simulink library "ddm"  (R2021b)
settings: Solver=VariableStepAuto  StartTime=0.0  StopTime=10.0  RelTol=1e-3
undefined symbols (not defined in the file or in its folder): ENUM_ADASACCSTA_ERROR, ENUM_ADASACCSTA_OFF, ENUM_ADASACCSTA_STANDBY, ENUM_ADASISASTA_OFF, ENUM_ALLOWMOV_ALLOWREADY, ENUM_APS, ENUM_BRKSTA_ERROR, ENUM_BRKSTA_OFF, ENUM_BRKSTA_ON, ENUM_BRKSW_INVALID, ENUM_BRKSW_OFF, ENUM_BRKSW_ON, ENUM_CHGPREACTERRSTA_OBCPRE, ENUM_DCDCFAULTSTA_ANYFAULTLV1, ENUM_DCDCFAULTSTA_ANYFAULTLV2, ENUM_DRIVETRAIN_AWD, ENUM_DRIVETRAIN_FWD, ENUM_DRIVETRAIN_RWD, ENUM_DRSEATSTA_INVALID, ENUM_EDUDRTSTA_NORMAL, ENUM_EPBSTA_APPLIED, ENUM_EPBSTA_RELEASED, ENUM_HVBATTREADYPRE_READY, ENUM_MCUWARN_LV0, ENUM_MCUWARN_LV1, ENUM_MCUWARN_LV2, ENUM_MCUWARN_LV3, ENUM_MCUWARN_NOERROR, ENUM_OBCFAULTSTA_ANYFAULT, ENUM_PAS_R2F2, ENUM_PDFAULT_BATTPDFAIL, ENUM_PDFAULT_DCDCDISABLE, ENUM_PDFAULT_MCUDISABLE, ENUM_PDFAULT_MCUDISCHRG, ENUM_POWERSTA_OFF, ENUM_POWERSTA_ON, ENUM_POWERSTA_READY, ENUM_POWERSTA_STANDBY, ENUM_PRESSINDI_LOW, ENUM_PUFAULT_BATTUPFAIL, ENUM_PUFAULT_DCDCENABLEFAIL, ENUM_PUFAULT_PRECHRGCHKFAIL, ENUM_PUFAULT_SAFETYCHKFAIL, ENUM_PUSTATE_COMPLETED, ENUM_PWRSTASW_OFF, ENUM_PWRSTASW_OFFA, ENUM_PWRSTASW_OFFCHVCHRG, ENUM_PWRSTASW_OFFCLVCHRG, ENUM_PWRSTASW_ON, ENUM_PWRSTASW_ONHVCHRG, ENUM_PWRSTASW_READY, ENUM_PWRSTASW_STANDBY, ENUM_RANGESTA_12IN, ENUM_SHIFTCOMMAND_D, ENUM_SHIFTCOMMAND_N, ENUM_SHIFTCOMMAND_P, ENUM_SHIFTCOMMAND_R, ENUM_VEHMALFUNLV_2ND, ENUM_VEHMALFUNLV_3RD, ENUM_VEHMALFUNLV_4TH ... (+835)
libraries: hcu_lib x750, $bdroot x12, simulink x5
(part 27 of 28)

== system ddm/DDM/DDM/VMC_DDM/MCU_Rr Signal Error/MCU_Rr Signal Error  ==
  note: Diagnostics and Fault Handling
  note: Fail Safe After Decision
  note: Release Condiction During Detection
  note: Release Condiction After Decision
  note: Test Pass Criteria
  note: Test Detection Criteria
  note: Fail Safe During Detection
  task_time_s : Inport
  VDDM_MCUF1NoComCFS_flg : Inport  Port=2
  VDDM_MCUF1RCErrCFS_flg : Inport  Port=3
  VDDM_MCUF1CSErrCFS_flg : Inport  Port=4
  No_CAN_BUS_OFF : Inport  Port=5
  VPMM_PowerSta_enum : Inport  Port=6
  VINP_MCUWarnR_enum : Inport  Port=7
  DTC_clear_request : Inport  Port=8
  Constant : Constant  Value=ENUM_POWERSTA_OFF
  Constant1 : Constant  Value=ENUM_POWERSTA_OFF
  Constant10 : Constant  Value=ENUM_MCUWARN_LV3
  Constant11 : Constant  Value=KDDM_RrMCUSigErrPassSW_flg
  Constant12 : Constant  Value=ENUM_POWERSTA_OFF
  Constant13 : Constant  Value=ENUM_POWERSTA_STANDBY
  Constant{5,14,18,22} (4 alike) : Constant  Value=TRUE
  Constant{2,15,20..21,23} (5 alike) : Constant  Value=FALSE
  Constant16 : Constant  Value=ENUM_MCUWARN_LV3
  Constant17 : Constant  Value=ENUM_MCUWARN_LV1
  Constant19 : Constant  Value=ENUM_MCUWARN_LV2
  Constant3 : Constant  Value=ENUM_MCUWARN_LV1
  Constant33 : Constant  Value=KDDM_RrMCUSigErrDetSW_flg
  Constant34 : Constant  Value=KDDM_RrMCUSigErrDTC_cnt
  Constant35 : Constant  Value=KDDM_RrMCUSigErrCFSSW_flg
  Constant36 : Constant  Value=KDDM_RrMCUSigErrDFSSW_flg
  Constant4 : Constant  Value=KDDM_RrMCUSigErrDetTO_ms
  Constant6 : Constant  Value=KDDM_RrMCUSigErrPassTO_ms
  Constant7 : Constant  Value=KDDM_RrMCUSigErrDTC_cnt
  Constant8 : Constant  Value=ENUM_MCUWARN_LV2
  Constant9 : Constant  Value=KDDM_RrMCUSigErrPassTO_ms
  DTC_Couter : hcu_lib/Basic_Blocks/DTC_Couter
  DTC_Info : hcu_lib/Basic_Blocks/DTC_Info
  Data Type Conversion1 : DataTypeConversion  OutDataTypeStr=uint8
  Equal : RelationalOperator  Operator=~=  OutDataTypeStr=boolean  RndMeth=Simplest
  Equal1 : RelationalOperator  Operator=~=  OutDataTypeStr=boolean  RndMeth=Simplest
  Equal{2,4..10} (8 alike) : RelationalOperator  Operator===  OutDataTypeStr=boolean  RndMeth=Simplest
  Equal3 : RelationalOperator  OutDataTypeStr=boolean  RndMeth=Simplest
  From1 : From  Commented=on  GotoTag=VDDM_RrMCUSigErrDFS_flg
  Gain : Gain  Gain=XX2KXX
  Gain1 : Gain  Gain=KXX2XX
  Goto7 : Goto  Commented=on  GotoTag=VDDM_EDriveSysErrVCUErr_flg
  Logical Operator{1,7..8,16,25} (5 alike) : Logic  Operator=OR  Inputs=3  AllPortsSameDT=off  OutDataTypeStr=boolean
  Logical Operator10 : Logic  Operator=OR  AllPortsSameDT=off  OutDataTypeStr=boolean
  Logical Operator{3,5,9,15} (4 alike) : Logic  AllPortsSameDT=off  OutDataTypeStr=boolean
  Logical Operator{4,6,17..18,20..22,24} (8 alike) : Logic  Operator=NOT  AllPortsSameDT=off  OutDataTypeStr=boolean
  Logical Operator19 : Logic  Inputs=3  AllPortsSameDT=off  OutDataTypeStr=boolean
  Logical Operator2 : Logic  Inputs=5  AllPortsSameDT=off  OutDataTypeStr=boolean
  Logical Operator23 : Logic  Inputs=5  AllPortsSameDT=off  OutDataTypeStr=boolean
  Relay : Relay  OnSwitchValue=ONE_INT  OffSwitchValue=ZERO_INT
  SR_Latch1 : hcu_lib/Basic_Blocks/SR_Latch
  SR_Latch4 : hcu_lib/Basic_Blocks/SR_Latch
  SR_Latch5 : hcu_lib/Basic_Blocks/SR_Latch
  Switch{,1..5} (6 alike) : Switch  Criteria=u2 ~= 0
  Terminator1 : Terminator
  Test Detection Criteria : hcu_lib/Basic_Blocks/Test Detection Criteria
  Timer1 : hcu_lib/Basic_Blocks/Timer
  Unit Delay2 : UnitDelay  SampleTime=-1  HasFrameUpgradeWarning=on
  VDDM_RrMCUSigErrCFS_flg : Outport
  VDDM_RrMCUSigErrDetDTC_raw32 : Outport  Port=2
  wires:
  Logical Operator15/1 -> DTC_Couter/2
  [DTC_clear_request] -> Logical Operator25/1, Logical Operator4/1
  Constant11/1 -> Logical Operator15/2
  [VDDM_RrMCUSigErrDet_flg] -> Logical Operator19/1
  Constant34/1 -> DTC_Couter/3
  [VDDM_RrMCUSigErrDTC_cnt] -> Relay/1
  Constant33/1 -> Logical Operator19/2
  [DTC_clear_request] -> Logical Operator7/3
  Logical Operator4/1 -> Logical Operator19/3
  Logical Operator10/1 -> SR_Latch5/2
  [VDDM_RrMCUSigErrDFSRls_flg] -> Logical Operator7/1
  DTC_Couter/2 -> Data Type Conversion1/1
  Data Type Conversion1/1 -> [VDDM_RrMCUSigErrDTC_cnt]
  Constant36/1 -> Logical Operator3/1
  SR_Latch5/1 -> Logical Operator5/1
  Logical Operator19/1 -> DTC_Couter/1
  SR_Latch4/1 -> Logical Operator3/2
  [VDDM_RrMCUSigErrCFSRls_flg] -> Logical Operator10/1
  [VDDM_RrMCUSigErrCFS_flg] -> Logical Operator7/2
  Constant35/1 -> Logical Operator5/2
  [VDDM_RrMCUSigErrCFSRls_flg] -> Logical Operator25/3
  Logical Operator7/1 -> SR_Latch4/2
  [VDDM_RrMCUSigErrPass_flg] -> Logical Operator25/2
  Logical Operator3/1 -> [VDDM_RrMCUSigErrDFS_flg]
  Logical Operator5/1 -> [VDDM_RrMCUSigErrCFS_flg]  "VDDM_RrMCUSigErrCFS_flg"
  [DTC_clear_request] -> Logical Operator10/2
  Logical Operator25/1 -> Logical Operator15/1
  DTC_Couter/1 -> SR_Latch5/1
  Relay/1 -> SR_Latch4/1
  DTC_Info/1 -> VDDM_RrMCUSigErrDetDTC_raw32/1  "VDDM_RrMCUSigErrDetDTC_raw32"
  [DTC_clear_request] -> DTC_Info/4
  [VDDM_RrMCUSigErrCFS_flg] -> DTC_Info/3
  [VDDM_RrMCUSigErrPass_flg] -> DTC_Info/2
  [VDDM_RrMCUSigErrDet_flg] -> DTC_Info/1
  Switch5/1 -> Test Detection Criteria/1
  Constant20/1 -> Switch5/1
  [DTC_clear_request] -> Switch5/2
  [VINP_MCUWarnR_enum] -> Equal10/1
  Constant16/1 -> Equal10/2
  [VINP_MCUWarnR_enum] -> Equal8/1
  Logical Operator1/1 -> Switch3/1
  Constant17/1 -> Equal8/2
  Equal8/1 -> Logical Operator1/1
  Equal9/1 -> Logical Operator1/2
  Equal10/1 -> Logical Operator1/3
  Constant19/1 -> Equal9/2
  [VINP_MCUWarnR_enum] -> Equal9/1
  Equal5/1 -> Logical Operator16/3
  Equal4/1 -> Logical Operator16/2
  Equal2/1 -> Logical Operator16/1
  Constant10/1 -> Equal5/2
  [VINP_MCUWarnR_enum] -> Equal5/1
  [VINP_MCUWarnR_enum] -> Equal4/1
  Constant8/1 -> Equal4/2
  Constant3/1 -> Equal2/2
  Constant9/1 -> Timer1/4
  Gain1/1 -> Timer1/3
  Test Detection Criteria/1 -> [VDDM_RrMCUSigErrDet_flg]  "VDDM_RrMCUSigErrDet_flg"
  Constant7/1 -> Test Detection Criteria/3
  Gain/1 -> Test Detection Criteria/4
  Constant4/1 -> Gain/1
  [task_time_s] -> Test Detection Criteria/2
  task_time_s/1 -> [task_time_s]  "task_time_s"
  Switch3/1 -> Logical Operator6/1, Timer1/2
  Constant1/1 -> Equal1/2
  [No_CAN_BUS_OFF] -> Logical Operator23/1
  [VDDM_MCUF1CSErrCFS_flg] -> Logical Operator24/1
  Logical Operator21/1 -> Logical Operator23/2
  Logical Operator24/1 -> Logical Operator23/4
  [VDDM_MCUF1RCErrCFS_flg] -> Logical Operator22/1
  Equal1/1 -> Logical Operator23/5
  Constant5/1 -> Switch3/3
  Logical Operator23/1 -> Switch3/2
  [VPMM_PowerSta_enum] -> Equal1/1
  [VDDM_MCUF1NoComCFS_flg] -> Logical Operator21/1
  Logical Operator22/1 -> Logical Operator23/3
  Logical Operator20/1 -> Logical Operator2/4
  Logical Operator18/1 -> Logical Operator2/3
  Logical Operator17/1 -> Logical Operator2/2
  [VINP_MCUWarnR_enum] -> Equal2/1
  Logical Operator16/1 -> Switch2/1
  [VDDM_MCUF1CSErrCFS_flg] -> Logical Operator20/1
  [VDDM_MCUF1RCErrCFS_flg] -> Logical Operator18/1
  [VDDM_MCUF1NoComCFS_flg] -> Logical Operator17/1
  Equal/1 -> Logical Operator2/5
  VINP_MCUWarnR_enum/1 -> [VINP_MCUWarnR_enum]
  No_CAN_BUS_OFF/1 -> [No_CAN_BUS_OFF]
  VDDM_MCUF1CSErrCFS_flg/1 -> [VDDM_MCUF1CSErrCFS_flg]
  VPMM_PowerSta_enum/1 -> [VPMM_PowerSta_enum]
  VDDM_MCUF1RCErrCFS_flg/1 -> [VDDM_MCUF1RCErrCFS_flg]
  DTC_clear_request/1 -> [DTC_clear_request]
  VDDM_MCUF1NoComCFS_flg/1 -> [VDDM_MCUF1NoComCFS_flg]
  Timer1/1 -> Equal3/1
  [VPMM_PowerSta_enum] -> Equal/1
  Logical Operator8/1 -> Switch4/2
  [VPMM_PowerSta_enum] -> Equal7/1
  Constant14/1 -> Switch4/1
  Constant2/1 -> Switch2/3
  Constant12/1 -> Equal6/2
  Unit Delay2/1 -> Equal6/1
  Constant/1 -> Equal/2
  Constant13/1 -> Equal7/2
  Logical Operator6/1 -> Timer1/1
  Logical Operator2/1 -> Switch2/2
  [DTC_clear_request] -> Logical Operator8/3
  [VDDM_xxx_flg] -> SR_Latch1/2
  [VDDM_RrMCUSigErrPass_flg] -> Logical Operator8/1
  [No_CAN_BUS_OFF] -> Logical Operator2/1
  Switch4/1 -> [VDDM_RrMCUSigErrCFSRls_flg]  "VDDM_RrMCUSigErrCFSRls_flg"
  Logical Operator9/1 -> Logical Operator8/2
  [VPMM_PowerSta_enum] -> Unit Delay2/1
  Constant6/1 -> Equal3/2
  Equal7/1 -> Logical Operator9/2
  Equal6/1 -> Logical Operator9/1
  [task_time_s] -> Gain1/1
  Equal3/1 -> SR_Latch1/1
  Constant15/1 -> Switch4/3
  [VDDM_RrMCUSigErrCFS_flg] -> VDDM_RrMCUSigErrCFS_flg/1
  From1/1 -> Terminator1/1
  SR_Latch1/1 -> [VDDM_RrMCUSigErrPass_flg]  "VDDM_RrMCUSigErrPass_flg"
  [VDDM_RrMCUSigErrPass_flg] -> Switch1/2
  [VDDM_RrMCUSigErrCFS_flg] -> Switch/2
  Constant18/1 -> Switch/1
  Switch/1 -> Goto7/1
  Constant21/1 -> Switch/3
  Switch1/1 -> [VDDM_RrMCUSigErrDFSRls_flg]
  Constant22/1 -> Switch1/1
  Constant23/1 -> Switch1/3
  Switch2/1 -> Switch5/3, [VDDM_xxx_flg]

== system ddm/DDM/DDM/VMC_DDM/MSA Malfunction /MSA Malfunction ==
  note: Diagnostics and Fault Handling
  note: Fail Safe After Decision
  note: Release Condiction During Detection
  note: Release Condiction After Decision
  note: Test Pass Criteria
  note: Test Detection Criteria
  note: Fail Safe During Detection
  task_time_s : Inport
  VDDM_BMSSigErrCFS_flg : Inport  Port=2
  VDDM_FrMCUSigErrCFS_flg : Inport  Port=3
  VDDM_RrMCUSigErrCFS_flg : Inport  Port=4
  VDDM_CCUSigErrCFS_flg : Inport  Port=5
  VDDM_ZoneSCPNoComCFS_flg : Inport  Port=6
  VDDM_MCUR1NoComCFS_flg : Inport  Port=7
  VDDM_MCUR1RCErrCFS_flg : Inport  Port=8
  VDDM_MCUR1CSErrCFS_flg : Inport  Port=9
  VDDM_MCUF1NoComCFS_flg : Inport  Port=10
  VDDM_MCUF1RCErrCFS_flg : Inport  Port=11
  VDDM_MCUF1CSErrCFS_flg : Inport  Port=12
  VDDM_ESC7NoComCFS_flg : Inport  Port=13
  VDDM_ESC7RCErrCFS_flg : Inport  Port=14
  VDDM_ESC7CSErrCFS_flg : Inport  Port=15
  VDDM_ESC1NoComCFS_flg : Inport  Port=16
  VDDM_ESC1RCErrCFS_flg : Inport  Port=17
  VDDM_ESC1CSErrCFS_flg : Inport  Port=18
  VDDM_ESC5NoComCFS_flg : Inport  Port=19
  VDDM_ESC5RCErrCFS_flg : Inport  Port=20
  VDDM_ESC5CSErrCFS_flg : Inport  Port=21
  No_CAN1_BUS_OFF : Inport  Port=22
  No_CAN3_BUS_OFF : Inport  Port=23
  No_CAN4_BUS_OFF : Inport  Port=24
  VPMM_PowerSta_enum : Inport  Port=25
  VINP_ZoneSpdCtrlMode_enum : Inport  Port=26
  DTC_clear_request : Inport  Port=27
  Constant1 : Constant  Value=ENUM_POWERSTA_READY
  Constant10 : Constant  Value=ENUM_ZONESPDCTRLMODE_LIM
  Constant11 : Constant  Value=KDDM_MSAMalfuncPassSW_flg
  Constant12 : Constant  Value=ENUM_POWERSTA_OFF
  Constant13 : Constant  Value=ENUM_POWERSTA_STANDBY
  Constant{5,14,18,22} (4 alike) : Constant  Value=TRUE
  Constant{2,15..16,21,23} (5 alike) : Constant  Value=FALSE
  Constant3 : Constant  Value=ENUM_ZONESPDCTRLMODE_LIM
  Constant33 : Constant  Value=KDDM_MSAMalfuncDetSW_flg
  Constant34 : Constant  Value=KDDM_MSAMalfuncDTC_cnt
  Constant35 : Constant  Value=KDDM_MSAMalfuncCFSSW_flg
  Constant36 : Constant  Value=KDDM_MSAMalfuncDFSSW_flg
  Constant4 : Constant  Value=KDDM_MSAMalfuncDetTO_ms
  Constant6 : Constant  Value=KDDM_MSAMalfuncPassTO_ms
  Constant7 : Constant  Value=KDDM_MSAMalfuncDTC_cnt
  Constant8 : Constant  Value=ENUM_POWERSTA_READY
  Constant9 : Constant  Value=KDDM_MSAMalfuncPassTO_ms
  DTC_Couter : hcu_lib/Basic_Blocks/DTC_Couter
  DTC_Info : hcu_lib/Basic_Blocks/DTC_Info
  Data Type Conversion1 : DataTypeConversion  OutDataTypeStr=uint8
  Equal{1..2,4..7} (6 alike) : RelationalOperator  Operator===  OutDataTypeStr=boolean  RndMeth=Simplest
  Equal3 : RelationalOperator  OutDataTypeStr=boolean  RndMeth=Simplest
  From1 : From  Commented=on  GotoTag=VDDM_MSAMalfuncDFS_flg
  Gain : Gain  Gain=XX2KXX
  Gain1 : Gain  Gain=KXX2XX
  Goto7 : Goto  Commented=on  GotoTag=VDDM_EDriveSysErrVCUErr_flg
  Logical Operator1 : Logic  Inputs=5  AllPortsSameDT=off  OutDataTypeStr=boolean
  Logical Operator12 : Logic  Operator=OR  Inputs=3  AllPortsSameDT=off  OutDataTypeStr=boolean
  Logical Operator{3,5,13,15} (4 alike) : Logic  AllPortsSameDT=off  OutDataTypeStr=boolean
  Logical Operator14 : Logic  Operator=OR  Inputs=20  AllPortsSameDT=off  OutDataTypeStr=boolean
  Logical Operator19 : Logic  Inputs=3  AllPortsSameDT=off  OutDataTypeStr=boolean
  Logical Operator2 : Logic  Inputs=5  AllPortsSameDT=off  OutDataTypeStr=boolean
  Logical Operator25 : Logic  Operator=OR  Inputs=3  AllPortsSameDT=off  OutDataTypeStr=boolean
  Logical Operator4 : Logic  Operator=OR  Inputs=20  AllPortsSameDT=off  OutDataTypeStr=boolean
  Logical Operator6 : Logic  Operator=NOT  AllPortsSameDT=off  OutDataTypeStr=boolean
  Logical Operator7 : Logic  Operator=OR  Inputs=3  AllPortsSameDT=off  OutDataTypeStr=boolean
  Logical Operator8 : Logic  Operator=NOT  AllPortsSameDT=off  OutDataTypeStr=boolean
  Logical Operator9 : Logic  Operator=OR  AllPortsSameDT=off  OutDataTypeStr=boolean
  Relay : Relay  OnSwitchValue=ONE_INT  OffSwitchValue=ZERO_INT
  SR_Latch1 : hcu_lib/Basic_Blocks/SR_Latch
  SR_Latch4 : hcu_lib/Basic_Blocks/SR_Latch
  SR_Latch5 : hcu_lib/Basic_Blocks/SR_Latch
  Switch{,1..5} (6 alike) : Switch  Criteria=u2 ~= 0
  Terminator1 : Terminator
  Test Detection Criteria : hcu_lib/Basic_Blocks/Test Detection Criteria
  Timer1 : hcu_lib/Basic_Blocks/Timer
  Unit Delay2 : UnitDelay  SampleTime=-1  HasFrameUpgradeWarning=on
  VDDM_MSAMalfuncCFS_flg : Outport
  VDDM_MSAMalfuncDetDTC_raw32 : Outport  Port=2
  wires:
  SR_Latch5/1 -> Logical Operator5/1
  [DTC_clear_request] -> Logical Operator7/3
  [DTC_clear_request] -> Logical Operator25/1, Logical Operator8/1
  Data Type Conversion1/1 -> [VDDM_MSAMalfuncDTC_cnt]  "VDDM_MSAMalfuncDTC_cnt"
  Logical Operator5/1 -> [VDDM_MSAMalfuncCFS_flg]  "VDDM_MSAMalfuncCFS_flg"
  Logical Operator8/1 -> Logical Operator19/3
  Constant35/1 -> Logical Operator5/2
  [VDDM_MSAMalfuncDTC_cnt] -> Relay/1
  SR_Latch4/1 -> Logical Operator3/2
  Logical Operator25/1 -> Logical Operator15/1
  Logical Operator15/1 -> DTC_Couter/2
  [VDDM_MSAMalfuncDFSRls_flg] -> Logical Operator7/1
  Logical Operator3/1 -> [VDDM_MSAMalfuncDFS_flg]
  Constant11/1 -> Logical Operator15/2
  [DTC_clear_request] -> Logical Operator9/2
  Logical Operator7/1 -> SR_Latch4/2
  Relay/1 -> SR_Latch4/1
  [VDDM_MSAMalfuncDet_flg] -> Logical Operator19/1
  DTC_Couter/2 -> Data Type Conversion1/1
  [VDDM_MSAMalfuncPass_flg] -> Logical Operator25/2
  [VDDM_MSAMalfuncCFSRls_flg] -> Logical Operator25/3
  Logical Operator19/1 -> DTC_Couter/1
  Constant34/1 -> DTC_Couter/3
  Constant33/1 -> Logical Operator19/2
  DTC_Couter/1 -> SR_Latch5/1
  [VDDM_MSAMalfuncCFSRls_flg] -> Logical Operator9/1
  Constant36/1 -> Logical Operator3/1
  [VDDM_MSAMalfuncCFS_flg] -> Logical Operator7/2
  Logical Operator9/1 -> SR_Latch5/2
  DTC_Info/1 -> VDDM_MSAMalfuncDetDTC_raw32/1  "VDDM_MSAMalfuncDetDTC_raw32"
  [DTC_clear_request] -> DTC_Info/4
  [VDDM_MSAMalfuncCFS_flg] -> DTC_Info/3
  [VDDM_MSAMalfuncPass_flg] -> DTC_Info/2
  [VDDM_MSAMalfuncDet_flg] -> DTC_Info/1
  Switch5/1 -> Test Detection Criteria/1
  Constant16/1 -> Switch5/1
  [DTC_clear_request] -> Switch5/2
  [VDDM_ESC5CSErrCFS_flg] -> Logical Operator4/20
  [VDDM_MCUR1CSErrCFS_flg] -> Logical Operator4/8
  [VDDM_ESC5NoComCFS_flg] -> Logical Operator4/18
  Logical Operator4/1 -> Switch3/1
  [VDDM_CCUSigErrCFS_flg] -> Logical Operator4/4
  [VDDM_MCUR1RCErrCFS_flg] -> Logical Operator4/7
  [VDDM_ESC1CSErrCFS_flg] -> Logical Operator4/17
  [VDDM_MCUF1NoComCFS_flg] -> Logical Operator4/9
  [VDDM_MCUR1NoComCFS_flg] -> Logical Operator4/6
  [VDDM_MCUF1CSErrCFS_flg] -> Logical Operator4/11
  [VDDM_MCUF1RCErrCFS_flg] -> Logical Operator4/10
  [VDDM_ESC7NoComCFS_flg] -> Logical Operator4/12
  [VDDM_ESC1NoComCFS_flg] -> Logical Operator4/15
  [VDDM_ESC7RCErrCFS_flg] -> Logical Operator4/13
  [VDDM_ESC5RCErrCFS_flg] -> Logical Operator4/19
  [VDDM_ESC7CSErrCFS_flg] -> Logical Operator4/14
  [VDDM_BMSSigErrCFS_flg] -> Logical Operator4/1
  [VDDM_FrMCUSigErrCFS_flg] -> Logical Operator4/2
  [VDDM_RrMCUSigErrCFS_flg] -> Logical Operator4/3
  [VDDM_ZoneSCPNoComCFS_flg] -> Logical Operator4/5
  [VDDM_ESC1RCErrCFS_flg] -> Logical Operator4/16
  [VDDM_ESC5CSErrCFS_flg] -> Logical Operator14/20
  [VDDM_ESC5RCErrCFS_flg] -> Logical Operator14/19
  [VDDM_ESC5NoComCFS_flg] -> Logical Operator14/18
  [VDDM_ESC1CSErrCFS_flg] -> Logical Operator14/17
  [VDDM_ESC1RCErrCFS_flg] -> Logical Operator14/16
  [VDDM_ESC1NoComCFS_flg] -> Logical Operator14/15
  [VDDM_ESC7CSErrCFS_flg] -> Logical Operator14/14
  [VDDM_ESC7RCErrCFS_flg] -> Logical Operator14/13
  [VDDM_ESC7NoComCFS_flg] -> Logical Operator14/12
  [VDDM_MCUF1CSErrCFS_flg] -> Logical Operator14/11
  [VDDM_MCUF1RCErrCFS_flg] -> Logical Operator14/10
  [VDDM_MCUF1NoComCFS_flg] -> Logical Operator14/9
  [VDDM_MCUR1CSErrCFS_flg] -> Logical Operator14/8
  [VDDM_MCUR1RCErrCFS_flg] -> Logical Operator14/7
  [VDDM_MCUR1NoComCFS_flg] -> Logical Operator14/6
  [VDDM_ZoneSCPNoComCFS_flg] -> Logical Operator14/5
  [VDDM_CCUSigErrCFS_flg] -> Logical Operator14/4
  [VDDM_RrMCUSigErrCFS_flg] -> Logical Operator14/3
  [VDDM_FrMCUSigErrCFS_flg] -> Logical Operator14/2
  [VDDM_BMSSigErrCFS_flg] -> Logical Operator14/1
  Logical Operator1/1 -> Switch3/2
  [No_CAN1_BUS_OFF] -> Logical Operator1/1
  [No_CAN3_BUS_OFF] -> Logical Operator1/2
  Equal4/1 -> Logical Operator1/5
  Equal5/1 -> Logical Operator1/4
  Constant8/1 -> Equal5/2
  Constant10/1 -> Equal4/2
  [VPMM_PowerSta_enum] -> Equal5/1
  [No_CAN4_BUS_OFF] -> Logical Operator1/3
  [VINP_ZoneSpdCtrlMode_enum] -> Equal4/1
  Equal1/1 -> Logical Operator2/5
  Constant3/1 -> Equal1/2
  [VINP_ZoneSpdCtrlMode_enum] -> Equal1/1
  [VPMM_PowerSta_enum] -> Equal2/1
  Constant1/1 -> Equal2/2
  Equal2/1 -> Logical Operator2/4
  [No_CAN4_BUS_OFF] -> Logical Operator2/3
  [No_CAN3_BUS_OFF] -> Logical Operator2/2
  Logical Operator14/1 -> Switch2/1
  VDDM_ESC5RCErrCFS_flg/1 -> [VDDM_ESC5RCErrCFS_flg]
  VDDM_ESC5CSErrCFS_flg/1 -> [VDDM_ESC5CSErrCFS_flg]
  VDDM_ESC5NoComCFS_flg/1 -> [VDDM_ESC5NoComCFS_flg]
  VDDM_ZoneSCPNoComCFS_flg/1 -> [VDDM_ZoneSCPNoComCFS_flg]
  task_time_s/1 -> [task_time_s]  "task_time_s"
  VINP_ZoneSpdCtrlMode_enum/1 -> [VINP_ZoneSpdCtrlMode_enum]
  No_CAN3_BUS_OFF/1 -> [No_CAN3_BUS_OFF]
  No_CAN1_BUS_OFF/1 -> [No_CAN1_BUS_OFF]
  VDDM_BMSSigErrCFS_flg/1 -> [VDDM_BMSSigErrCFS_flg]
  VDDM_ESC7NoComCFS_flg/1 -> [VDDM_ESC7NoComCFS_flg]
  VDDM_ESC7CSErrCFS_flg/1 -> [VDDM_ESC7CSErrCFS_flg]
  VPMM_PowerSta_enum/1 -> [VPMM_PowerSta_enum]
  No_CAN4_BUS_OFF/1 -> [No_CAN4_BUS_OFF]
  VDDM_ESC7RCErrCFS_flg/1 -> [VDDM_ESC7RCErrCFS_flg]
  VDDM_RrMCUSigErrCFS_flg/1 -> [VDDM_RrMCUSigErrCFS_flg]
  VDDM_CCUSigErrCFS_flg/1 -> [VDDM_CCUSigErrCFS_flg]
  VDDM_FrMCUSigErrCFS_flg/1 -> [VDDM_FrMCUSigErrCFS_flg]
  VDDM_MCUF1RCErrCFS_flg/1 -> [VDDM_MCUF1RCErrCFS_flg]
  VDDM_ESC1NoComCFS_flg/1 -> [VDDM_ESC1NoComCFS_flg]
  DTC_clear_request/1 -> [DTC_clear_request]
  VDDM_MCUR1RCErrCFS_flg/1 -> [VDDM_MCUR1RCErrCFS_flg]
  VDDM_MCUR1CSErrCFS_flg/1 -> [VDDM_MCUR1CSErrCFS_flg]
  VDDM_ESC1RCErrCFS_flg/1 -> [VDDM_ESC1RCErrCFS_flg]
  VDDM_ESC1CSErrCFS_flg/1 -> [VDDM_ESC1CSErrCFS_flg]
  VDDM_MCUF1CSErrCFS_flg/1 -> [VDDM_MCUF1CSErrCFS_flg]
  VDDM_MCUF1NoComCFS_flg/1 -> [VDDM_MCUF1NoComCFS_flg]
  VDDM_MCUR1NoComCFS_flg/1 -> [VDDM_MCUR1NoComCFS_flg]
  [VDDM_MSAMalfuncPass_flg] -> Logical Operator12/1
  Constant12/1 -> Equal6/2
  Constant13/1 -> Equal7/2
  Equal6/1 -> Logical Operator13/1
  Logical Operator13/1 -> Logical Operator12/2
  Equal7/1 -> Logical Operator13/2
  Unit Delay2/1 -> Equal6/1
  [VPMM_PowerSta_enum] -> Equal7/1
  [VPMM_PowerSta_enum] -> Unit Delay2/1
  Constant9/1 -> Timer1/4
  Gain1/1 -> Timer1/3
  Test Detection Criteria/1 -> [VDDM_MSAMalfuncDet_flg]  "VDDM_MSAMalfuncDet_flg"
  Constant7/1 -> Test Detection Criteria/3
  Gain/1 -> Test Detection Criteria/4
  Constant4/1 -> Gain/1
  [task_time_s] -> Test Detection Criteria/2
  Switch3/1 -> Logical Operator6/1, Timer1/2
  Constant5/1 -> Switch3/3
  Timer1/1 -> Equal3/1
  Logical Operator12/1 -> Switch4/2
  Constant14/1 -> Switch4/1
  Constant2/1 -> Switch2/3
  Logical Operator6/1 -> Timer1/1
  Logical Operator2/1 -> Switch2/2
  [DTC_clear_request] -> Logical Operator12/3
  [VDDM_xxx_flg] -> SR_Latch1/2
  [No_CAN1_BUS_OFF] -> Logical Operator2/1
  Switch4/1 -> [VDDM_MSAMalfuncCFSRls_flg]  "VDDM_MSAMalfuncCFSRls_flg"
  Constant6/1 -> Equal3/2
  [task_time_s] -> Gain1/1
  Equal3/1 -> SR_Latch1/1
  Constant15/1 -> Switch4/3
  [VDDM_MSAMalfuncCFS_flg] -> VDDM_MSAMalfuncCFS_flg/1
  From1/1 -> Terminator1/1
  SR_Latch1/1 -> [VDDM_MSAMalfuncPass_flg]  "VDDM_MSAMalfuncPass_flg"
  [VDDM_MSAMalfuncPass_flg] -> Switch1/2
  [VDDM_MSAMalfuncCFS_flg] -> Switch/2
  Constant18/1 -> Switch/1
  Switch/1 -> Goto7/1
  Constant21/1 -> Switch/3
  Switch1/1 -> [VDDM_MSAMalfuncDFSRls_flg]
  Constant22/1 -> Switch1/1
  Constant23/1 -> Switch1/3
  Switch2/1 -> Switch5/3, [VDDM_xxx_flg]

== system ddm/DDM/DDM/VMC_DDM/ZoneSCP/ZoneSCP Lost Com ==
  note: Diagnostics and Fault Handling
  note: Fail Safe During Detection
  note: Test Detection Criteria
  note: Release Condiction After Decision
  note: Test Pass Criteria
  note: Release Condiction During Detection
  note: Fail Safe After Decision
  task_time_s : Inport
  VDDM_ZoneSCPNoCom_flg : Inport  Port=2
  No_CAN_BUS_OFF : Inport  Port=3
  VPMM_PowerSta_enum : Inport  Port=4
  VINP_VehSpeed_kph : Inport  Port=5
  DTC_clear_request : Inport  Port=6
  Constant : Constant  Value=ENUM_POWERSTA_OFF
  Constant1 : Constant  Value=KDDM_ZoneSCPNoComCFSRls_kph
  Constant12 : Constant  Value=ENUM_POWERSTA_OFF
  Constant13 : Constant  Value=ENUM_POWERSTA_STANDBY
  Constant{7,14,18,22} (4 alike) : Constant  Value=TRUE
  Constant{2,8,15,21,23} (5 alike) : Constant  Value=FALSE
  Constant3 : Constant  Value=KDDM_ZoneSCPNoComDFSRls_kph
  Constant31 : Constant  Value=KDDM_ZoneSCPNoComDFSSW_flg
  Constant4 : Constant  Value=KDDM_ZoneSCPNoComCFSSW_flg
  Constant40 : Constant  Value=KDDM_ZoneSCPNoComDTC_cnt
  Constant41 : Constant  Value=KDDM_ZoneSCPNoComDetTO_ms
  Constant45 : Constant  Value=KDDM_ZoneSCPNoComPassSW_flg
  Constant46 : Constant  Value=KDDM_ZoneSCPNoComDetSW_flg
  Constant48 : Constant  Value=KDDM_ZoneSCPNoComDTC_cnt
  Constant5 : Constant  Value=ENUM_POWERSTA_OFF
  Constant6 : Constant  Value=KDDM_ZoneSCPNoComPassTO_ms
  Constant9 : Constant  Value=KDDM_ZoneSCPNoComPassTO_ms
  DTC_Couter : hcu_lib/Basic_Blocks/DTC_Couter
  DTC_Info : hcu_lib/Basic_Blocks/DTC_Info
  Data Type Conversion1 : DataTypeConversion  OutDataTypeStr=uint8
  Equal : RelationalOperator  Operator=~=  OutDataTypeStr=boolean  RndMeth=Simplest
  Equal1 : RelationalOperator  Operator=<=  OutDataTypeStr=boolean  RndMeth=Simplest
  Equal2 : RelationalOperator  Operator=~=  OutDataTypeStr=boolean  RndMeth=Simplest
  Equal3 : RelationalOperator  OutDataTypeStr=boolean  RndMeth=Simplest
  Equal4 : RelationalOperator  Operator=<=  OutDataTypeStr=boolean  RndMeth=Simplest
  Equal6 : RelationalOperator  Operator===  OutDataTypeStr=boolean  RndMeth=Simplest
  Equal7 : RelationalOperator  Operator===  OutDataTypeStr=boolean  RndMeth=Simplest
  From6 : From  Commented=on  GotoTag=VDDM_EDriveSysErrVCUErr_flg
  Gain : Gain  Gain=XX2KXX
  Gain1 : Gain  Gain=KXX2XX
  Goto7 : Goto  Commented=on  GotoTag=VDDM_EDriveSysErrVCUErr_flg
  Logical Operator{1..2,4..5,9,12,15,18} (8 alike) : Logic  AllPortsSameDT=off  OutDataTypeStr=boolean
  Logical Operator10 : Logic  Operator=OR  AllPortsSameDT=off  OutDataTypeStr=boolean
  Logical Operator19 : Logic  Inputs=3  AllPortsSameDT=off  OutDataTypeStr=boolean
  Logical Operator21 : Logic  Operator=OR  Inputs=3  AllPortsSameDT=off  OutDataTypeStr=boolean
  Logical Operator3 : Logic  Operator=OR  Inputs=3  AllPortsSameDT=off  OutDataTypeStr=boolean
  Logical Operator6 : Logic  Operator=NOT  AllPortsSameDT=off  OutDataTypeStr=boolean
  Logical Operator7 : Logic  Operator=NOT  AllPortsSameDT=off  OutDataTypeStr=boolean
  Logical Operator8 : Logic  Operator=OR  Inputs=3  AllPortsSameDT=off  OutDataTypeStr=boolean
  Relay : Relay  OnSwitchValue=ONE_INT  OffSwitchValue=ZERO_INT
  SR_Latch1 : hcu_lib/Basic_Blocks/SR_Latch
  SR_Latch3 : hcu_lib/Basic_Blocks/SR_Latch
  SR_Latch4 : hcu_lib/Basic_Blocks/SR_Latch
  Switch{,1..5} (6 alike) : Switch  Criteria=u2 ~= 0
  Terminator : Terminator
  Test Detection Criteria : hcu_lib/Basic_Blocks/Test Detection Criteria
  Timer1 : hcu_lib/Basic_Blocks/Timer
  Unit Delay2 : UnitDelay  SampleTime=-1  HasFrameUpgradeWarning=on
  VDDM_ZoneSCPNoComDFS_flg : Outport
  VDDM_ZoneSCPNoComCFS_flg : Outport  Port=2
  VDDM_ZoneSCPNoComDTC_raw32 : Outport  Port=3
  wires:
  Logical Operator3/1 -> Logical Operator15/1
  Logical Operator7/1 -> Logical Operator19/3
  [DTC_clear_request] -> Logical Operator21/3
  Constant48/1 -> DTC_Couter/3
  Logical Operator10/1 -> SR_Latch4/2
  DTC_Couter/2 -> Data Type Conversion1/1
  [DTC_clear_request] -> Logical Operator10/2
  SR_Latch3/1 -> Logical Operator12/2
  [DTC_clear_request] -> Logical Operator3/1, Logical Operator7/1
  Logical Operator15/1 -> DTC_Couter/2
  SR_Latch4/1 -> Logical Operator18/1
  Constant45/1 -> Logical Operator15/2
  Constant31/1 -> Logical Operator12/1
  [VDDM_ZoneSCPNoComDet_flg] -> Logical Operator19/1
  Logical Operator21/1 -> SR_Latch3/2
  Logical Operator12/1 -> [VDDM_ZoneSCPNoComDFS_flg]  "VDDM_ZoneSCPNoComDFS_flg"
  Relay/1 -> SR_Latch3/1
  [VDDM_ZoneSCPNoComCFS_flg] -> Logical Operator21/2
  Data Type Conversion1/1 -> [VDDM_ZoneSCPNoComDTC_cnt]
  [VDDM_ZoneSCPNoComCFSRls_flg] -> Logical Operator3/3
  Logical Operator18/1 -> [VDDM_ZoneSCPNoComCFS_flg]  "VDDM_ZoneSCPNoComCFS_flg"
  [VDDM_ZoneSCPNoComCFSRls_flg] -> Logical Operator10/1
  Constant4/1 -> Logical Operator18/2
  [VDDM_ZoneSCPNoComDTC_cnt] -> Relay/1
  [VDDM_ZoneSCPNoComPass_flg] -> Logical Operator3/2
  [VDDM_ZoneSCPNoComDFSRls_flg] -> Logical Operator21/1
  Constant46/1 -> Logical Operator19/2
  DTC_Couter/1 -> SR_Latch4/1
  Logical Operator19/1 -> DTC_Couter/1
  DTC_Info/1 -> VDDM_ZoneSCPNoComDTC_raw32/1  "VDDM_ZoneSCPNoComDTC_raw32"
  [DTC_clear_request] -> DTC_Info/4
  [VDDM_ZoneSCPNoComCFS_flg] -> DTC_Info/3
  [VDDM_ZoneSCPNoComPass_flg] -> DTC_Info/2
  [VDDM_ZoneSCPNoComDet_flg] -> DTC_Info/1
  Switch5/1 -> Test Detection Criteria/1
  [DTC_clear_request] -> Switch5/2
  Constant8/1 -> Switch5/1
  Equal4/1 -> Logical Operator1/2
  [VDDM_ZoneSCPNoComPass_flg] -> Logical Operator1/1
  Logical Operator1/1 -> Switch1/2
  [VINP_VehSpeed_kph] -> Equal4/1
  Constant3/1 -> Equal4/2
  Constant1/1 -> Equal1/2
  [VINP_VehSpeed_kph] -> Equal1/1
  Equal1/1 -> Logical Operator5/2
  Gain1/1 -> Timer1/3
  Constant9/1 -> Timer1/4
  task_time_s/1 -> [task_time_s]  "task_time_s"
  Constant40/1 -> Test Detection Criteria/3
  Constant6/1 -> Equal3/2
  SR_Latch1/1 -> [VDDM_ZoneSCPNoComPass_flg]  "VDDM_ZoneSCPNoComPass_flg"
  Gain/1 -> Test Detection Criteria/4
  Equal/1 -> Logical Operator2/2
  [VDDM_ZoneSCPNoComPass_flg] -> Logical Operator5/1
  Equal2/1 -> Logical Operator4/2
  [No_CAN_BUS_OFF] -> Logical Operator4/1
  Logical Operator9/1 -> Logical Operator8/2
  Logical Operator8/1 -> Switch4/2
  [VPMM_PowerSta_enum] -> Equal7/1
  [VPMM_PowerSta_enum] -> Equal2/1
  [VDDM_ZoneSCPNoCom_flg] -> Switch3/1
  Switch2/1 -> Switch5/3, [VDDM_xxx_flg]
  Constant/1 -> Equal/2
  Switch3/1 -> Timer1/2, Logical Operator6/1
  [VPMM_PowerSta_enum] -> Equal/1
  Switch4/1 -> [VDDM_ZoneSCPNoComCFSRls_flg]  "VDDM_ZoneSCPNoComCFSRls_flg"
  Constant41/1 -> Gain/1
  [task_time_s] -> Test Detection Criteria/2
  Test Detection Criteria/1 -> [VDDM_ZoneSCPNoComDet_flg]  "VDDM_ZoneSCPNoComDet_flg"
  Logical Operator2/1 -> Switch2/2
  Constant23/1 -> Switch1/3
  Timer1/1 -> Equal3/1
  Constant21/1 -> Switch/3
  Equal7/1 -> Logical Operator9/2
  [VDDM_ZoneSCPNoCom_flg] -> Switch2/1
  Logical Operator5/1 -> Logical Operator8/1
  Constant7/1 -> Switch3/3
  Logical Operator4/1 -> Switch3/2
  Constant14/1 -> Switch4/1
  Constant2/1 -> Switch2/3
  Constant12/1 -> Equal6/2
  Unit Delay2/1 -> Equal6/1
  [DTC_clear_request] -> Logical Operator8/3
  Constant5/1 -> Equal2/2
  Switch/1 -> Goto7/1
  Switch1/1 -> [VDDM_ZoneSCPNoComDFSRls_flg]  "VDDM_ZoneSCPNoComDFSRls_flg"
  Equal3/1 -> SR_Latch1/1
  Constant18/1 -> Switch/1
  Constant13/1 -> Equal7/2
  Equal6/1 -> Logical Operator9/1
  [task_time_s] -> Gain1/1
  Constant15/1 -> Switch4/3
  [VPMM_PowerSta_enum] -> Unit Delay2/1
  [VDDM_ZoneSCPNoComCFS_flg] -> Switch/2
  [No_CAN_BUS_OFF] -> Logical Operator2/1
  [VDDM_xxx_flg] -> SR_Latch1/2
  Constant22/1 -> Switch1/1
  Logical Operator6/1 -> Timer1/1
  From6/1 -> Terminator/1
  [VDDM_ZoneSCPNoComDFS_flg] -> VDDM_ZoneSCPNoComDFS_flg/1
  [VDDM_ZoneSCPNoComCFS_flg] -> VDDM_ZoneSCPNoComCFS_flg/1
  VDDM_ZoneSCPNoCom_flg/1 -> [VDDM_ZoneSCPNoCom_flg]
  VINP_VehSpeed_kph/1 -> [VINP_VehSpeed_kph]
  No_CAN_BUS_OFF/1 -> [No_CAN_BUS_OFF]
  DTC_clear_request/1 -> [DTC_clear_request]
  VPMM_PowerSta_enum/1 -> [VPMM_PowerSta_enum]

== system ddm/DDM/DDM/PMM/Brake switch signal abnormal/Brake switch signal abnormal/SR_Latch1 ==
  set : Inport
  reset : Inport  Port=2
  Logical Operator : Logic  AllPortsSameDT=off  OutDataTypeStr=boolean
  Logical Operator1 : Logic  Operator=NOT  AllPortsSameDT=off  OutDataTypeStr=boolean
  Switch1 : Switch  Criteria=u2 ~= 0  Threshold=0.5
      settings: AttributesFormatString=<Criteria=%<Criteria>>
  Switch2 : Switch  Criteria=u2 ~= 0  Threshold=0.5
      settings: AttributesFormatString=<Criteria=%<Criteria>>
  Unit Delay : UnitDelay  SampleTime=-1  HasFrameUpgradeWarning=on
  latched : Outport
  wires:
  Logical Operator1/1 -> Switch2/1, Logical Operator/2
  Logical Operator/1 -> Switch1/2
  Switch2/1 -> Switch1/3
  Unit Delay/1 -> Switch2/3
  reset/1 -> Logical Operator1/1, Switch2/2
  set/1 -> Logical Operator/1, Switch1/1
  Switch1/1 -> latched/1, Unit Delay/1

== system ddm/DDM/DDM/PMM/Brake switch signal abnormal/Brake switch signal abnormal and no backup signal/SR_Latch1 ==
  set : Inport
  reset : Inport  Port=2
  Logical Operator : Logic  AllPortsSameDT=off  OutDataTypeStr=boolean
  Logical Operator1 : Logic  Operator=NOT  AllPortsSameDT=off  OutDataTypeStr=boolean
  Switch1 : Switch  Criteria=u2 ~= 0  Threshold=0.5
      settings: AttributesFormatString=<Criteria=%<Criteria>>
  Switch2 : Switch  Criteria=u2 ~= 0  Threshold=0.5
      settings: AttributesFormatString=<Criteria=%<Criteria>>
  Unit Delay : UnitDelay  SampleTime=-1  HasFrameUpgradeWarning=on
  latched : Outport
  wires:
  Logical Operator1/1 -> Switch2/1, Logical Operator/2
  Logical Operator/1 -> Switch1/2
  Switch2/1 -> Switch1/3
  Unit Delay/1 -> Switch2/3
  reset/1 -> Logical Operator1/1, Switch2/2
  set/1 -> Logical Operator/1, Switch1/1
  Switch1/1 -> latched/1, Unit Delay/1

== system ddm/DDM/DDM/PMM/Comm err/FDC lost communication with EPAS2/SR_Latch1 ==
  set : Inport
  reset : Inport  Port=2
  Logical Operator : Logic  AllPortsSameDT=off  OutDataTypeStr=boolean
  Logical Operator1 : Logic  Operator=NOT  AllPortsSameDT=off  OutDataTypeStr=boolean
  Switch1 : Switch  Criteria=u2 ~= 0  Threshold=0.5
      settings: AttributesFormatString=<Criteria=%<Criteria>>
  Switch2 : Switch  Criteria=u2 ~= 0  Threshold=0.5
      settings: AttributesFormatString=<Criteria=%<Criteria>>
  Unit Delay : UnitDelay  SampleTime=-1  HasFrameUpgradeWarning=on
  latched : Outport
  wires:
  Switch1/1 -> Unit Delay/1, latched/1
  set/1 -> Switch1/1, Logical Operator/1
  reset/1 -> Switch2/2, Logical Operator1/1
  Unit Delay/1 -> Switch2/3
  Switch2/1 -> Switch1/3
  Logical Operator/1 -> Switch1/2
  Logical Operator1/1 -> Logical Operator/2, Switch2/1

== system ddm/DDM/DDM/PMM/Comm err/The CAN signal between VCU and ABM1 is discontinuous/SR_Latch1 ==
  set : Inport
  reset : Inport  Port=2
  Logical Operator : Logic  AllPortsSameDT=off  OutDataTypeStr=boolean
  Logical Operator1 : Logic  Operator=NOT  AllPortsSameDT=off  OutDataTypeStr=boolean
  Switch1 : Switch  Criteria=u2 ~= 0  Threshold=0.5
      settings: AttributesFormatString=<Criteria=%<Criteria>>
  Switch2 : Switch  Criteria=u2 ~= 0  Threshold=0.5
      settings: AttributesFormatString=<Criteria=%<Criteria>>
  Unit Delay : UnitDelay  SampleTime=-1  HasFrameUpgradeWarning=on
  latched : Outport
  wires:
  Logical Operator1/1 -> Switch2/1, Logical Operator/2
  Logical Operator/1 -> Switch1/2
  Switch2/1 -> Switch1/3
  Unit Delay/1 -> Switch2/3
  reset/1 -> Logical Operator1/1, Switch2/2
  set/1 -> Logical Operator/1, Switch1/1
  Switch1/1 -> latched/1, Unit Delay/1

== system ddm/DDM/DDM/PMM/Comm err/The CAN signal between VCU and ABM1 is incomplete/SR_Latch1 ==
  set : Inport
  reset : Inport  Port=2
  Logical Operator : Logic  AllPortsSameDT=off  OutDataTypeStr=boolean
  Logical Operator1 : Logic  Operator=NOT  AllPortsSameDT=off  OutDataTypeStr=boolean
  Switch1 : Switch  Criteria=u2 ~= 0  Threshold=0.5
      settings: AttributesFormatString=<Criteria=%<Criteria>>
  Switch2 : Switch  Criteria=u2 ~= 0  Threshold=0.5
      settings: AttributesFormatString=<Criteria=%<Criteria>>
  Unit Delay : UnitDelay  SampleTime=-1  HasFrameUpgradeWarning=on
  latched : Outport
  wires:
  Logical Operator1/1 -> Switch2/1, Logical Operator/2
  Logical Operator/1 -> Switch1/2
  Switch2/1 -> Switch1/3
  Unit Delay/1 -> Switch2/3
  reset/1 -> Logical Operator1/1, Switch2/2
  set/1 -> Logical Operator/1, Switch1/1
  Switch1/1 -> latched/1, Unit Delay/1

== system ddm/DDM/DDM/PMM/Comm err/The CAN signal between VCU and BMS1 is discontinuous/SR_Latch1 ==
  set : Inport
  reset : Inport  Port=2
  Logical Operator : Logic  AllPortsSameDT=off  OutDataTypeStr=boolean
  Logical Operator1 : Logic  Operator=NOT  AllPortsSameDT=off  OutDataTypeStr=boolean
  Switch1 : Switch  Criteria=u2 ~= 0  Threshold=0.5
      settings: AttributesFormatString=<Criteria=%<Criteria>>
  Switch2 : Switch  Criteria=u2 ~= 0  Threshold=0.5
      settings: AttributesFormatString=<Criteria=%<Criteria>>
  Unit Delay : UnitDelay  SampleTime=-1  HasFrameUpgradeWarning=on
  latched : Outport
  wires:
  Logical Operator1/1 -> Switch2/1, Logical Operator/2
  Logical Operator/1 -> Switch1/2
  Switch2/1 -> Switch1/3
  Unit Delay/1 -> Switch2/3
  reset/1 -> Logical Operator1/1, Switch2/2
  set/1 -> Logical Operator/1, Switch1/1
  Switch1/1 -> latched/1, Unit Delay/1

== system ddm/DDM/DDM/PMM/Comm err/The CAN signal between VCU and BMS1 is incomplete/SR_Latch1 ==
  set : Inport
  reset : Inport  Port=2
  Logical Operator : Logic  AllPortsSameDT=off  OutDataTypeStr=boolean
  Logical Operator1 : Logic  Operator=NOT  AllPortsSameDT=off  OutDataTypeStr=boolean
  Switch1 : Switch  Criteria=u2 ~= 0  Threshold=0.5
      settings: AttributesFormatString=<Criteria=%<Criteria>>
  Switch2 : Switch  Criteria=u2 ~= 0  Threshold=0.5
      settings: AttributesFormatString=<Criteria=%<Criteria>>
  Unit Delay : UnitDelay  SampleTime=-1  HasFrameUpgradeWarning=on
  latched : Outport
  wires:
  Logical Operator1/1 -> Switch2/1, Logical Operator/2
  Logical Operator/1 -> Switch1/2
  Switch2/1 -> Switch1/3
  Unit Delay/1 -> Switch2/3
  reset/1 -> Logical Operator1/1, Switch2/2
  set/1 -> Logical Operator/1, Switch1/1
  Switch1/1 -> latched/1, Unit Delay/1

== system ddm/DDM/DDM/PMM/Comm err/The CAN signal between VCU and BMS6 is discontinuous/SR_Latch1 ==
  set : Inport
  reset : Inport  Port=2
  Logical Operator : Logic  AllPortsSameDT=off  OutDataTypeStr=boolean
  Logical Operator1 : Logic  Operator=NOT  AllPortsSameDT=off  OutDataTypeStr=boolean
  Switch1 : Switch  Criteria=u2 ~= 0  Threshold=0.5
      settings: AttributesFormatString=<Criteria=%<Criteria>>
  Switch2 : Switch  Criteria=u2 ~= 0  Threshold=0.5
      settings: AttributesFormatString=<Criteria=%<Criteria>>
  Unit Delay : UnitDelay  SampleTime=-1  HasFrameUpgradeWarning=on
  latched : Outport
  wires:
  Logical Operator1/1 -> Switch2/1, Logical Operator/2
  Logical Operator/1 -> Switch1/2
  Switch2/1 -> Switch1/3
  Unit Delay/1 -> Switch2/3
  reset/1 -> Logical Operator1/1, Switch2/2
  set/1 -> Logical Operator/1, Switch1/1
  Switch1/1 -> latched/1, Unit Delay/1

== system ddm/DDM/DDM/PMM/Comm err/The CAN signal between VCU and BMS6 is incomplete/SR_Latch1 ==
  set : Inport
  reset : Inport  Port=2
  Logical Operator : Logic  AllPortsSameDT=off  OutDataTypeStr=boolean
  Logical Operator1 : Logic  Operator=NOT  AllPortsSameDT=off  OutDataTypeStr=boolean
  Switch1 : Switch  Criteria=u2 ~= 0  Threshold=0.5
      settings: AttributesFormatString=<Criteria=%<Criteria>>
  Switch2 : Switch  Criteria=u2 ~= 0  Threshold=0.5
      settings: AttributesFormatString=<Criteria=%<Criteria>>
  Unit Delay : UnitDelay  SampleTime=-1  HasFrameUpgradeWarning=on
  latched : Outport
  wires:
  Logical Operator1/1 -> Switch2/1, Logical Operator/2
  Logical Operator/1 -> Switch1/2
  Switch2/1 -> Switch1/3
  Unit Delay/1 -> Switch2/3
  reset/1 -> Logical Operator1/1, Switch2/2
  set/1 -> Logical Operator/1, Switch1/1
  Switch1/1 -> latched/1, Unit Delay/1

== system ddm/DDM/DDM/PMM/Comm err/The CAN signal between VCU and CCU1 is discontinuous/SR_Latch1 ==
  set : Inport
  reset : Inport  Port=2
  Logical Operator : Logic  AllPortsSameDT=off  OutDataTypeStr=boolean
  Logical Operator1 : Logic  Operator=NOT  AllPortsSameDT=off  OutDataTypeStr=boolean
  Switch1 : Switch  Criteria=u2 ~= 0  Threshold=0.5
      settings: AttributesFormatString=<Criteria=%<Criteria>>
  Switch2 : Switch  Criteria=u2 ~= 0  Threshold=0.5
      settings: AttributesFormatString=<Criteria=%<Criteria>>
  Unit Delay : UnitDelay  SampleTime=-1  HasFrameUpgradeWarning=on
  latched : Outport
  wires:
  Logical Operator1/1 -> Switch2/1, Logical Operator/2
  Logical Operator/1 -> Switch1/2
  Switch2/1 -> Switch1/3
  Unit Delay/1 -> Switch2/3
  reset/1 -> Logical Operator1/1, Switch2/2
  set/1 -> Logical Operator/1, Switch1/1
  Switch1/1 -> latched/1, Unit Delay/1

== system ddm/DDM/DDM/PMM/Comm err/The CAN signal between VCU and CCU1 is incomplete/SR_Latch1 ==
  set : Inport
  reset : Inport  Port=2
  Logical Operator : Logic  AllPortsSameDT=off  OutDataTypeStr=boolean
  Logical Operator1 : Logic  Operator=NOT  AllPortsSameDT=off  OutDataTypeStr=boolean
  Switch1 : Switch  Criteria=u2 ~= 0  Threshold=0.5
      settings: AttributesFormatString=<Criteria=%<Criteria>>
  Switch2 : Switch  Criteria=u2 ~= 0  Threshold=0.5
      settings: AttributesFormatString=<Criteria=%<Criteria>>
  Unit Delay : UnitDelay  SampleTime=-1  HasFrameUpgradeWarning=on
  latched : Outport
  wires:
  Logical Operator1/1 -> Switch2/1, Logical Operator/2
  Logical Operator/1 -> Switch1/2
  Switch2/1 -> Switch1/3
  Unit Delay/1 -> Switch2/3
  reset/1 -> Logical Operator1/1, Switch2/2
  set/1 -> Logical Operator/1, Switch1/1
  Switch1/1 -> latched/1, Unit Delay/1

== system ddm/DDM/DDM/PMM/Comm err/The CAN signal between VCU and CCU2 is discontinuous/SR_Latch1 ==
  set : Inport
  reset : Inport  Port=2
  Logical Operator : Logic  AllPortsSameDT=off  OutDataTypeStr=boolean
  Logical Operator1 : Logic  Operator=NOT  AllPortsSameDT=off  OutDataTypeStr=boolean
  Switch1 : Switch  Criteria=u2 ~= 0  Threshold=0.5
      settings: AttributesFormatString=<Criteria=%<Criteria>>
  Switch2 : Switch  Criteria=u2 ~= 0  Threshold=0.5
      settings: AttributesFormatString=<Criteria=%<Criteria>>
  Unit Delay : UnitDelay  SampleTime=-1  HasFrameUpgradeWarning=on
  latched : Outport
  wires:
  Logical Operator1/1 -> Switch2/1, Logical Operator/2
  Logical Operator/1 -> Switch1/2
  Switch2/1 -> Switch1/3
  Unit Delay/1 -> Switch2/3
  reset/1 -> Logical Operator1/1, Switch2/2
  set/1 -> Logical Operator/1, Switch1/1
  Switch1/1 -> latched/1, Unit Delay/1

== system ddm/DDM/DDM/PMM/Comm err/The CAN signal between VCU and CCU2 is incomplete/SR_Latch1 ==
  set : Inport
  reset : Inport  Port=2
  Logical Operator : Logic  AllPortsSameDT=off  OutDataTypeStr=boolean
  Logical Operator1 : Logic  Operator=NOT  AllPortsSameDT=off  OutDataTypeStr=boolean
  Switch1 : Switch  Criteria=u2 ~= 0  Threshold=0.5
      settings: AttributesFormatString=<Criteria=%<Criteria>>
  Switch2 : Switch  Criteria=u2 ~= 0  Threshold=0.5
      settings: AttributesFormatString=<Criteria=%<Criteria>>
  Unit Delay : UnitDelay  SampleTime=-1  HasFrameUpgradeWarning=on
  latched : Outport
  wires:
  Logical Operator1/1 -> Switch2/1, Logical Operator/2
  Logical Operator/1 -> Switch1/2
  Switch2/1 -> Switch1/3
  Unit Delay/1 -> Switch2/3
  reset/1 -> Logical Operator1/1, Switch2/2
  set/1 -> Logical Operator/1, Switch1/1
  Switch1/1 -> latched/1, Unit Delay/1

== system ddm/DDM/DDM/PMM/Comm err/VCU lost communication with ABM1/SR_Latch1 ==
  set : Inport
  reset : Inport  Port=2
  Logical Operator : Logic  AllPortsSameDT=off  OutDataTypeStr=boolean
  Logical Operator1 : Logic  Operator=NOT  AllPortsSameDT=off  OutDataTypeStr=boolean
  Switch1 : Switch  Criteria=u2 ~= 0  Threshold=0.5
      settings: AttributesFormatString=<Criteria=%<Criteria>>
  Switch2 : Switch  Criteria=u2 ~= 0  Threshold=0.5
      settings: AttributesFormatString=<Criteria=%<Criteria>>
  Unit Delay : UnitDelay  SampleTime=-1  HasFrameUpgradeWarning=on
  latched : Outport
  wires:
  Logical Operator1/1 -> Switch2/1, Logical Operator/2
  Logical Operator/1 -> Switch1/2
  Switch2/1 -> Switch1/3
  Unit Delay/1 -> Switch2/3
  reset/1 -> Logical Operator1/1, Switch2/2
  set/1 -> Logical Operator/1, Switch1/1
  Switch1/1 -> latched/1, Unit Delay/1

== system ddm/DDM/DDM/PMM/Comm err/VCU lost communication with BMS1/SR_Latch1 ==
  set : Inport
  reset : Inport  Port=2
  Logical Operator : Logic  AllPortsSameDT=off  OutDataTypeStr=boolean
  Logical Operator1 : Logic  Operator=NOT  AllPortsSameDT=off  OutDataTypeStr=boolean
  Switch1 : Switch  Criteria=u2 ~= 0  Threshold=0.5
      settings: AttributesFormatString=<Criteria=%<Criteria>>
  Switch2 : Switch  Criteria=u2 ~= 0  Threshold=0.5
      settings: AttributesFormatString=<Criteria=%<Criteria>>
  Unit Delay : UnitDelay  SampleTime=-1  HasFrameUpgradeWarning=on
  latched : Outport
  wires:
  Logical Operator1/1 -> Switch2/1, Logical Operator/2
  Logical Operator/1 -> Switch1/2
  Switch2/1 -> Switch1/3
  Unit Delay/1 -> Switch2/3
  reset/1 -> Logical Operator1/1, Switch2/2
  set/1 -> Logical Operator/1, Switch1/1
  Switch1/1 -> latched/1, Unit Delay/1

== system ddm/DDM/DDM/PMM/Comm err/VCU lost communication with BMS6/SR_Latch1 ==
  set : Inport
  reset : Inport  Port=2
  Logical Operator : Logic  AllPortsSameDT=off  OutDataTypeStr=boolean
  Logical Operator1 : Logic  Operator=NOT  AllPortsSameDT=off  OutDataTypeStr=boolean
  Switch1 : Switch  Criteria=u2 ~= 0  Threshold=0.5
      settings: AttributesFormatString=<Criteria=%<Criteria>>
  Switch2 : Switch  Criteria=u2 ~= 0  Threshold=0.5
      settings: AttributesFormatString=<Criteria=%<Criteria>>
  Unit Delay : UnitDelay  SampleTime=-1  HasFrameUpgradeWarning=on
  latched : Outport
  wires:
  Logical Operator1/1 -> Switch2/1, Logical Operator/2
  Logical Operator/1 -> Switch1/2
  Switch2/1 -> Switch1/3
  Unit Delay/1 -> Switch2/3
  reset/1 -> Logical Operator1/1, Switch2/2
  set/1 -> Logical Operator/1, Switch1/1
  Switch1/1 -> latched/1, Unit Delay/1

== system ddm/DDM/DDM/PMM/Comm err/VCU lost communication with CCU1/SR_Latch1 ==
  set : Inport
  reset : Inport  Port=2
  Logical Operator : Logic  AllPortsSameDT=off  OutDataTypeStr=boolean
  Logical Operator1 : Logic  Operator=NOT  AllPortsSameDT=off  OutDataTypeStr=boolean
  Switch1 : Switch  Criteria=u2 ~= 0  Threshold=0.5
      settings: AttributesFormatString=<Criteria=%<Criteria>>
  Switch2 : Switch  Criteria=u2 ~= 0  Threshold=0.5
      settings: AttributesFormatString=<Criteria=%<Criteria>>
  Unit Delay : UnitDelay  SampleTime=-1  HasFrameUpgradeWarning=on
  latched : Outport
  wires:
  Logical Operator1/1 -> Switch2/1, Logical Operator/2
  Logical Operator/1 -> Switch1/2
  Switch2/1 -> Switch1/3
  Unit Delay/1 -> Switch2/3
  reset/1 -> Logical Operator1/1, Switch2/2
  set/1 -> Logical Operator/1, Switch1/1
  Switch1/1 -> latched/1, Unit Delay/1

== system ddm/DDM/DDM/PMM/Comm err/VCU lost communication with CCU2/SR_Latch1 ==
  set : Inport
  reset : Inport  Port=2
  Logical Operator : Logic  AllPortsSameDT=off  OutDataTypeStr=boolean
  Logical Operator1 : Logic  Operator=NOT  AllPortsSameDT=off  OutDataTypeStr=boolean
  Switch1 : Switch  Criteria=u2 ~= 0  Threshold=0.5
      settings: AttributesFormatString=<Criteria=%<Criteria>>
  Switch2 : Switch  Criteria=u2 ~= 0  Threshold=0.5
      settings: AttributesFormatString=<Criteria=%<Criteria>>
  Unit Delay : UnitDelay  SampleTime=-1  HasFrameUpgradeWarning=on
  latched : Outport
  wires:
  Logical Operator1/1 -> Switch2/1, Logical Operator/2
  Logical Operator/1 -> Switch1/2
  Switch2/1 -> Switch1/3
  Unit Delay/1 -> Switch2/3
  reset/1 -> Logical Operator1/1, Switch2/2
  set/1 -> Logical Operator/1, Switch1/1
  Switch1/1 -> latched/1, Unit Delay/1

== system ddm/DDM/DDM/PMM/Fault level/Fault level 1 subsystem error/SR_Latch1 ==
  set : Inport
  reset : Inport  Port=2
  Logical Operator : Logic  AllPortsSameDT=off  OutDataTypeStr=boolean
  Logical Operator1 : Logic  Operator=NOT  AllPortsSameDT=off  OutDataTypeStr=boolean
  Switch1 : Switch  Criteria=u2 ~= 0  Threshold=0.5
      settings: AttributesFormatString=<Criteria=%<Criteria>>
  Switch2 : Switch  Criteria=u2 ~= 0  Threshold=0.5
      settings: AttributesFormatString=<Criteria=%<Criteria>>
  Unit Delay : UnitDelay  SampleTime=-1  HasFrameUpgradeWarning=on
  latched : Outport
  wires:
  Logical Operator1/1 -> Switch2/1, Logical Operator/2
  Logical Operator/1 -> Switch1/2
  Switch2/1 -> Switch1/3
  Unit Delay/1 -> Switch2/3
  reset/1 -> Logical Operator1/1, Switch2/2
  set/1 -> Logical Operator/1, Switch1/1
  Switch1/1 -> latched/1, Unit Delay/1

== system ddm/DDM/DDM/PMM/Fault level/Fault level 2 subsystem error/SR_Latch1 ==
  set : Inport
  reset : Inport  Port=2
  Logical Operator : Logic  AllPortsSameDT=off  OutDataTypeStr=boolean
  Logical Operator1 : Logic  Operator=NOT  AllPortsSameDT=off  OutDataTypeStr=boolean
  Switch1 : Switch  Criteria=u2 ~= 0  Threshold=0.5
      settings: AttributesFormatString=<Criteria=%<Criteria>>
  Switch2 : Switch  Criteria=u2 ~= 0  Threshold=0.5
      settings: AttributesFormatString=<Criteria=%<Criteria>>
  Unit Delay : UnitDelay  SampleTime=-1  HasFrameUpgradeWarning=on
  latched : Outport
  wires:
  Logical Operator1/1 -> Switch2/1, Logical Operator/2
  Logical Operator/1 -> Switch1/2
  Switch2/1 -> Switch1/3
  Unit Delay/1 -> Switch2/3
  reset/1 -> Logical Operator1/1, Switch2/2
  set/1 -> Logical Operator/1, Switch1/1
  Switch1/1 -> latched/1, Unit Delay/1

== system ddm/DDM/DDM/PMM/Fault level/Fault level 3 subsystem error/SR_Latch1 ==
  set : Inport
  reset : Inport  Port=2
  Logical Operator : Logic  AllPortsSameDT=off  OutDataTypeStr=boolean
  Logical Operator1 : Logic  Operator=NOT  AllPortsSameDT=off  OutDataTypeStr=boolean
  Switch1 : Switch  Criteria=u2 ~= 0  Threshold=0.5
      settings: AttributesFormatString=<Criteria=%<Criteria>>
  Switch2 : Switch  Criteria=u2 ~= 0  Threshold=0.5
      settings: AttributesFormatString=<Criteria=%<Criteria>>
  Unit Delay : UnitDelay  SampleTime=-1  HasFrameUpgradeWarning=on
  latched : Outport
  wires:
  Logical Operator1/1 -> Switch2/1, Logical Operator/2
  Logical Operator/1 -> Switch1/2
  Switch2/1 -> Switch1/3
  Unit Delay/1 -> Switch2/3
  reset/1 -> Logical Operator1/1, Switch2/2
  set/1 -> Logical Operator/1, Switch1/1
  Switch1/1 -> latched/1, Unit Delay/1

== system ddm/DDM/DDM/PMM/Fault level/Fault level 4 subsystem error/SR_Latch1 ==
  set : Inport
  reset : Inport  Port=2
  Logical Operator : Logic  AllPortsSameDT=off  OutDataTypeStr=boolean
  Logical Operator1 : Logic  Operator=NOT  AllPortsSameDT=off  OutDataTypeStr=boolean
  Switch1 : Switch  Criteria=u2 ~= 0  Threshold=0.5
      settings: AttributesFormatString=<Criteria=%<Criteria>>
  Switch2 : Switch  Criteria=u2 ~= 0  Threshold=0.5
      settings: AttributesFormatString=<Criteria=%<Criteria>>
  Unit Delay : UnitDelay  SampleTime=-1  HasFrameUpgradeWarning=on
  latched : Outport
  wires:
  Logical Operator1/1 -> Switch2/1, Logical Operator/2
  Logical Operator/1 -> Switch1/2
  Switch2/1 -> Switch1/3
  Unit Delay/1 -> Switch2/3
  reset/1 -> Logical Operator1/1, Switch2/2
  set/1 -> Logical Operator/1, Switch1/1
  Switch1/1 -> latched/1, Unit Delay/1
